simulink model "potenlab"  (R2024b)
settings: Solver=FixedStepAuto  StartTime=0.0  StopTime=inf  FixedStep=1  RelTol=1e-3  EnableMultiTasking=on
libraries: stm32f4xxblockslib x3, spsCurrentMeasurementLib x1, spsDCVoltageSourceLib x1, simulink x1, spsGroundLib x1, spsIdealSwitchLib x1, spsSeriesRLCBranchLib x1, spspowerguiLib x1
(part 2 of 2)

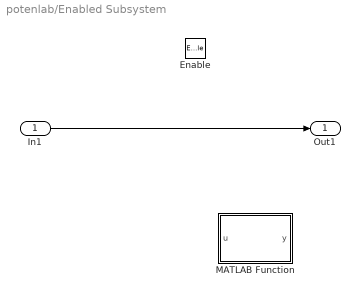
== system potenlab/Enabled Subsystem ==
  In1 : Inport
  Enable : EnablePort
  MATLAB Function : MATLAB Function  TreatAsAtomicUnit=on
  Out1 : Outport
  wires:
  In1/1 -> Out1/1

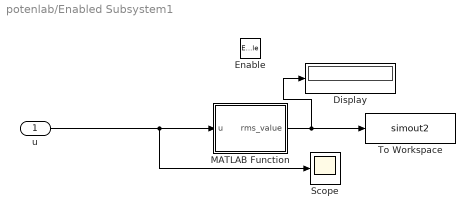
== system potenlab/Enabled Subsystem1 ==
  u : Inport
  Enable : EnablePort
  Display : Display
  MATLAB Function : MATLAB Function  TreatAsAtomicUnit=on
  Scope : Scope
  To Workspace : ToWorkspace  VariableName=simout2  SaveFormat=Timeseries  SampleTime=-1
  wires:
  u/1 -> Scope/1, MATLAB Function/1(u)
  MATLAB Function/1(rms_value) -> Display/1, To Workspace/1

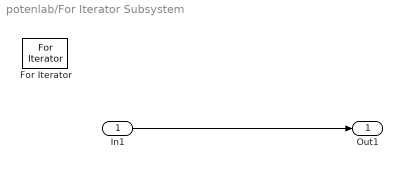
== system potenlab/For Iterator Subsystem ==
  In1 : Inport
  For Iterator : ForIterator
  Out1 : Outport
  wires:
  In1/1 -> Out1/1

== matlab function potenlab/Enabled Subsystem1/MATLAB Function ==
  data: u input; rms_value output
function rms_value = fcn(u)
    % Get the size of input data u
    n = length(u);  % Determine how many elements are in u
    
    % Initialize an array to store the 1000 data points
    persistent data_array;  % Use persistent to store data across function calls
    persistent count;       % To keep track of how many data points have been stored
    
    if isempty(data_array)
        data_array = zeros(500, 1);  % Preallocate space for 1000 data points
        count = 0;                    % Initialize the count
    end
    
    % Loop through each element of the input data and store it
    for i = 1:n
        if count < 500
            count = count + 1;
            data_array(count) = u(i);  % Store the data
        end
    end
    
    % Once 1000 data points have been stored, calculate the RMS
    if count == 500
        % Calculate the RMS value
        rms_value = sqrt(mean(data_array.^2));
        
        % Reset the count and data_array if needed for continuous calculations
        count = 0;
        data_array = zeros(500, 1);
    else
        rms_value = NaN;  % Output NaN until 1000 points have been collected
    end
end

== matlab function potenlab/Enabled Subsystem/MATLAB Function ==
  data: u input; y output
function y = fcn(u)

for i = 1:length(10):
y = u;

== stateflow chart potenlab/Chart ==
  state initial
    entry:
    time=0;
    outputvolt;
    output= 0;
  state State
    entry:
    output = 1;
    during:
    time = time + 0.001;
    exit:
    output = 0;
    time = 0;
  (default) -> initial
  initial -> State : [input == 1]
  State -> initial : [time > 1]
  data: input input; outputvolt input; output output; time local

== stateflow chart potenlab/Schmitt Trigger ==
  state initial
    input;
    output=0;
  state High
    entry:
    output=1;
  (default) -> initial
  initial -> High : [input>=2]
  High -> initial : [input<1]
  data: input input; output output
